simulink model "ballbeam_sim"  (R2015a)
settings: Solver=ode45  StartTime=0.0  StopTime=200  RelTol=1e-3
InitFcn:
  | param
undefined symbols (not defined in the file or in its folder): ballbeam_ctrl, drawBallBeam, P
settings Model: Creator=beard  LastModifiedBy=beard
settings DataIOCC: SignalLoggingSaveFormat=ModelDataLogs
settings OptimizationCC: ExpressionDepthLimit=2147483647  InitFltsAndDblsToZero=on
settings DebuggingCC: UnderspecifiedInitializationDetection=Classic  MergeDetectMultiDrivingBlocksExec=none  SolverPrmCheckMsg=warning  FcnCallInpInsideContextMsg=UseLocalSettings  StateNameClashWarn=warning
settings GRTTargetCC: CombineOutputUpdateFcns=off  GRTInterface=on

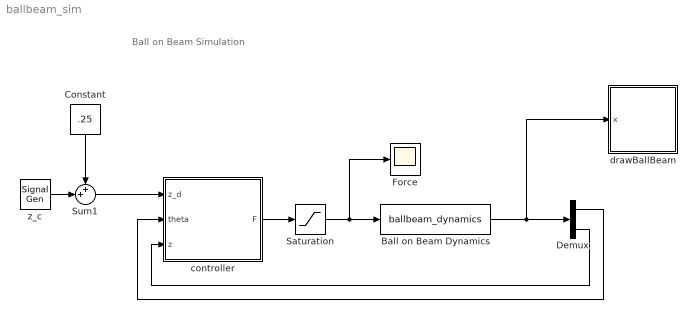
== system ballbeam_sim ==
  note: Ball on Beam Simulation
  Ball on Beam Dynamics : S-Function  FunctionName=ballbeam_dynamics  Parameters=AP
  Constant : Constant  Value=.25
  Demux : Demux  Outputs=2
  Force : Scope
      settings: YMin=-2.5  YMax=15  SaveName=ScopeData2
  Saturation : Saturate  UpperLimit=P.Fmax  LowerLimit=-P.Fmax
  Sum1 : Sum  Inputs=++|
  controller : Subsystem
  drawBallBeam : Subsystem
      mask Display: image(imread('tv.jpg'))
  z_c : SignalGenerator  WaveForm=square  Amplitude=.15  Frequency=.02
  wires:
  Ball on Beam Dynamics/1 -> drawBallBeam/1(x), Demux/1
  z_c/1 -> Sum1/2
  Sum1/1 -> controller/1(z_d)
  Constant/1 -> Sum1/1
  Saturation/1 -> Force/1, Ball on Beam Dynamics/1
  controller/1(F) -> Saturation/1
  Demux/2 -> controller/3(z)
  Demux/1 -> controller/2(theta)

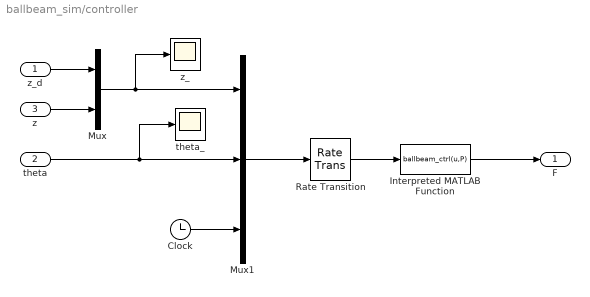
== system ballbeam_sim/controller ==
  z_d : Inport
  theta : Inport  Port=2
  z : Inport  Port=3
  Clock : Clock
  Interpreted MATLAB Function : MATLABFcn  MATLABFcn=ballbeam_ctrl(u,P)  OutputDimensions=1
  Mux : Mux  Inputs=2
  Mux1 : Mux  Inputs=3
  Rate Transition : RateTransition  OutPortSampleTime=P.Ts
  theta_ : Scope
      settings: TimeRange=100  YMin=-2  YMax=1.5
  z_ : Scope
      settings: TimeRange=100  YMin=0  YMax=0.475
  F : Outport
  wires:
  Mux1/1 -> Rate Transition/1
  Interpreted MATLAB Function/1 -> F/1
  Rate Transition/1 -> Interpreted MATLAB Function/1
  theta/1 -> theta_/1, Mux1/2
  z_d/1 -> Mux/1
  z/1 -> Mux/2
  Mux/1 -> z_/1, Mux1/1
  Clock/1 -> Mux1/3

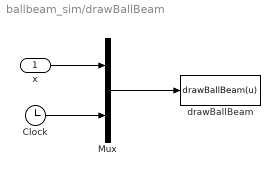
== system ballbeam_sim/drawBallBeam ==
  x : Inport
  Clock : Clock
  Mux : Mux  Inputs=2
  drawBallBeam : MATLABFcn  MATLABFcn=drawBallBeam(u)  OutputDimensions=0  SampleTime=0.1
  wires:
  Mux/1 -> drawBallBeam/1
  x/1 -> Mux/1
  Clock/1 -> Mux/2
